simulink subsystem "Tutorial_Simulink_4_subsystem"  (R2023b)
settings: Solver=VariableStepAuto  StartTime=0.0  StopTime=10.0  RelTol=1e-3
settings Model: Creator=admin  LastModifiedBy=admin

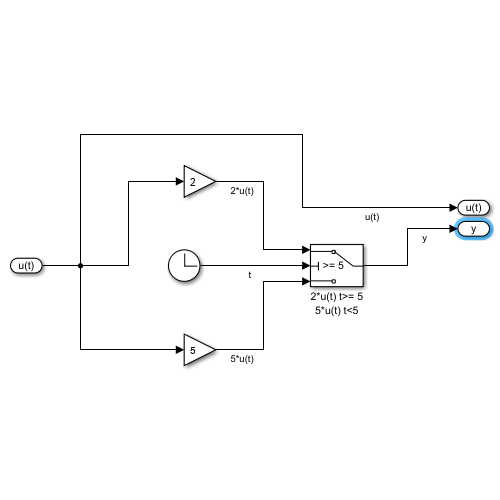
[thumbnail: Simulink's stored preview of the top-level diagram]
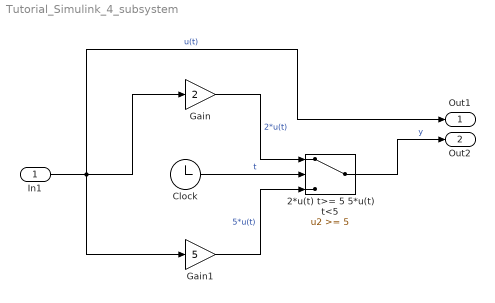
== system Tutorial_Simulink_4_subsystem ==
  In1 : Inport
  2*u(t) t>= 5 5*u(t) t<5 : Switch  Threshold=5  SaturateOnIntegerOverflow=off  InputSameDT=off
  Clock : Clock
  Gain : Gain  Gain=2
  Gain1 : Gain  Gain=5
  Out1 : Outport
  Out2 : Outport  Port=2
  wires:
  In1/1 -> Out1/1, Gain/1, Gain1/1  "u(t)"
  Gain/1 -> 2*u(t) t>= 5 5*u(t) t<5/1  "2*u(t)"
  2*u(t) t>= 5 5*u(t) t<5/1 -> Out2/1  "y"
  Gain1/1 -> 2*u(t) t>= 5 5*u(t) t<5/3  "5*u(t)"
  Clock/1 -> 2*u(t) t>= 5 5*u(t) t<5/2  "t"
